simulink model "inverter"  (R2026a)
settings: Solver=VariableStepAuto  StopTime=0.5
libraries: fl_lib x18, nesl_utility x8, ee_lib x2
settings Model: Creator=bilgehan  LastModifiedBy=bilgehan
settings DataIOCC: SaveState=on

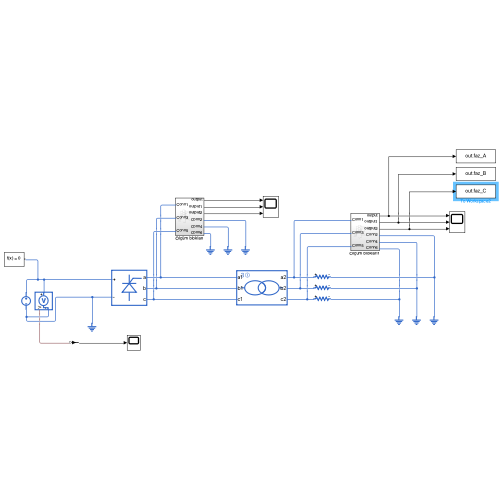
[thumbnail: Simulink's stored preview of the top-level diagram]
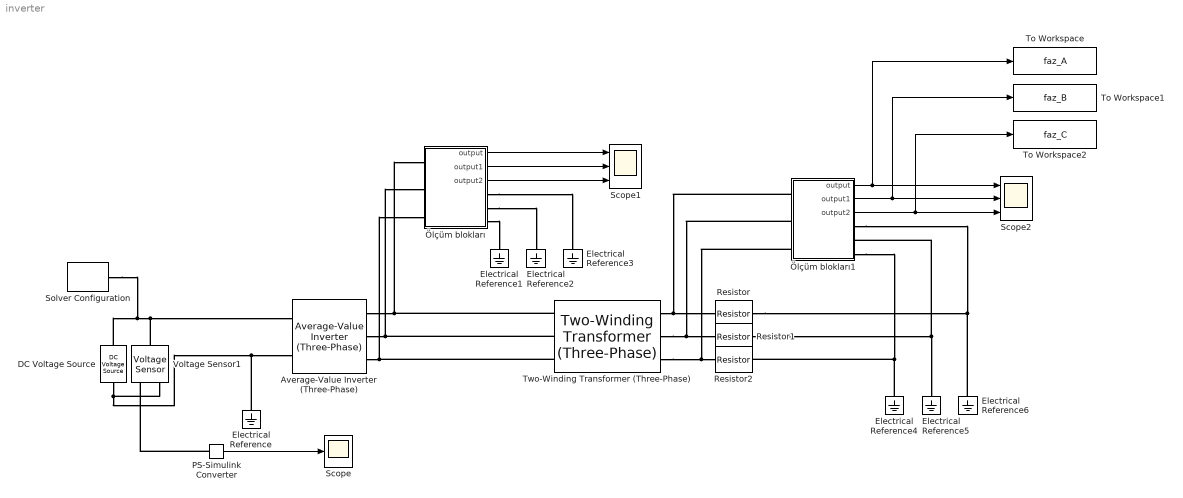
== system inverter ==
  Average-Value Inverter (Three-Phase) : ee_lib/Semiconductors & Converters/Converters/Average-Value Inverter (Three-Phase)  port_option=ee.enum.threePhasePort.expanded  FRated=50 Hz  PhaseShift=0 deg  voltage_ratio=sqrt(6) / pi  Pfixed=1e3 W  v_on=100 V  v_off=75 V
  DC Voltage Source : fl_lib/Electrical/Electrical Sources/DC Voltage Source  v0=400 V
  Electrical Reference{,1..6} (7 alike) : fl_lib/Electrical/Electrical Elements/Electrical Reference
  PS-Simulink Converter : nesl_utility/PS-Simulink Converter  PhysicalDomain=network_engine_domain  SubClassName=ps_output  LeftPortType=input  RightPortType=output  PseudoPeriodic=off  Frequencies=[]  VectorFormat=inherit  Unit=inherit  AffineConversion=off
  Resistor : fl_lib/Electrical/Electrical Elements/Resistor  R=50 Ohm  i_specify=off  i_priority=None  i=0 A  i_nominal_specify=off  i_nominal_value=1  i_nominal_unit=A  v_specify=off  v_priority=None  v=0 V  v_nominal_specify=off  v_nominal_value=1  v_nominal_unit=V
  Resistor1 : fl_lib/Electrical/Electrical Elements/Resistor  R=50 Ohm  i_specify=off  i_priority=None  i=0 A  i_nominal_specify=off  i_nominal_value=1  i_nominal_unit=A  v_specify=off  v_priority=None  v=0 V  v_nominal_specify=off  v_nominal_value=1  v_nominal_unit=V
  Resistor2 : fl_lib/Electrical/Electrical Elements/Resistor  R=50 Ohm  i_specify=off  i_priority=None  i=0 A  i_nominal_specify=off  i_nominal_value=1  i_nominal_unit=A  v_specify=off  v_priority=None  v=0 V  v_nominal_specify=off  v_nominal_value=1  v_nominal_unit=V
  Scope : Scope
      settings: ActiveDisplayYMinimum=-118.30988508385255  ActiveDisplayYMaximum=518.30988605563437
  Scope1 : Scope  NumInputPorts=3
      settings: ActiveDisplayYMinimum=-118.30987454094273  ActiveDisplayYMaximum=518.30988273667788
  Scope2 : Scope  NumInputPorts=3
      settings: ActiveDisplayYMinimum=-402.70817553940793  ActiveDisplayYMaximum=402.70749472920392  DataLoggingVariableName=trafo_out
  Solver Configuration : nesl_utility/Solver Configuration  PhysicalDomain=network_engine_domain  SubClassName=solver  LeftPortType=input  RightPortType=generic  Tones=[]  Harmonics=[]  SimulateNoise=off  Profile=off  UseLocalSampling=off  EnableSwitchedLinearOptims=on  FrequencyDomain=off  UseCCode=off  RelTol=0.001  AbsTol=0.001  MinStep=1e-09  ToWorkspace=off  RevertToSquareIcSolve=off  NumHomotopyIterations=100  PhasorMode=off  PhasorModeNumHarmonics=1  ConsistencySolver=NEWTON_XTOL_AFTER_FTOL  CanonicalOrdering=CANONICAL  OptimizeIntermediates=OPTIMIZED  IndexReductionMethod=DerivativeReplacement  DoDC=off  ResidualTolerance=1e-09  ConsistencyTolSource=GLOBAL  ConsistencyAbsTol=0.001  ConsistencyRelTol=0.001  ConsistencyTolFactor=0.001  UseLocalSolver=off  LocalSolverChoice=NE_BACKWARD_EULER_ADVANCER  ResolveIndetEquations=on  FunctionEvalNumThread=1  LocalSolverSampleTime=0.001  DoFixedCost=off  MaxNonlinIter=3  MaxModeIter=2  ComputeImpulses=off  ImpulseIterations=2  LinearAlgebra=auto  LinearAlgebraNumThread=0  EquationFormulation=NE_TIME_EF  DelaysMemoryBudget=1024  AutomaticFiltering=on  FilteringTimeConstant=0.001  PartitionStorageMethod=AS_NEEDED  PartitionMemoryBudget=1024  PartitionMethod=ROBUST  MultibodyUseLocalSolver=off  MultibodyLocalSolverChoice=ODE1  MultibodyLocalSolverSampleTime=0.001
  To Workspace : ToWorkspace  VariableName=faz_A  SampleTime=-1
  To Workspace1 : ToWorkspace  VariableName=faz_B  SampleTime=-1
  To Workspace2 : ToWorkspace  VariableName=faz_C  SampleTime=-1
  Two-Winding Transformer (Three-Phase) : ee_lib/Passive/Transformers/Two-Winding Transformer (Three-Phase)  SRated=3250 A*V  FRated=50 Hz  Winding1Connection=ee.enum.windingconnection.Y  VRated1=311 V  Winding2Connection=ee.enum.windingconnection.Y  VRated2=400 V  CoreType=ee.enum.coretype.threelimb  pu_Rw1=0.002  pu_Rw2=0.01  leakage_reactance_option=ee.enum.transformer_leakage.include  pu_Xl1=0.05  pu_Xl2=0.05  magnetizing_resistance_option=ee.enum.transformer_magnetizingResistance.exclude  pu_Rm=500  magnetizing_reactance_option=ee.enum.transformer_magnetizingReactance.exclude  saturation_option=ee.enum.transformer_saturation.exclude  pu_Xm=500  current_data=[0, .002, 1, 2]  magnetic_flux_data=[0, 1.2, 1.5, 1.51]  pu_X0=0.5  i1_specify=off  i1_priority=None  i1=[0, 0, 0] A  i1_nominal_specify=off  i1_nominal_value=1  i1_nominal_unit=A  i2_specify=off  i2_priority=None  i2=[0, 0, 0] A  i2_nominal_specify=off  i2_nominal_value=1  i2_nominal_unit=A  phi_specify=off  phi_priority=None  phi=[0, 0, 0]  phi_nominal_specify=off  phi_nominal_value=1  phi_nominal_unit=1
  Voltage Sensor1 : fl_lib/Electrical/Electrical Sensors/Voltage Sensor
  Ölçüm blokları : Subsystem
  Ölçüm blokları1 : Subsystem
  wires:
  PS-Simulink Converter/1 -> Scope/1
  Ölçüm blokları/1(output) -> Scope1/1
  Ölçüm blokları/2(output1) -> Scope1/2
  Ölçüm blokları/3(output2) -> Scope1/3
  Ölçüm blokları1/2(output1) -> To Workspace1/1, Scope2/2
  Ölçüm blokları1/3(output2) -> To Workspace2/1, Scope2/3
  Ölçüm blokları1/1(output) -> To Workspace/1, Scope2/1
  connections:
  DC Voltage Source/LConn1 -- Solver Configuration/RConn1 -- Average-Value Inverter (Three-Phase)/LConn1 -- Voltage Sensor1/LConn1
  DC Voltage Source/RConn1 -- Voltage Sensor1/RConn2 -- Average-Value Inverter (Three-Phase)/LConn2 -- Electrical Reference/LConn1
  Average-Value Inverter (Three-Phase)/RConn1 -- Two-Winding Transformer (Three-Phase)/LConn1 -- Ölçüm blokları/LConn1
  Average-Value Inverter (Three-Phase)/RConn2 -- Two-Winding Transformer (Three-Phase)/LConn2 -- Ölçüm blokları/LConn2
  Average-Value Inverter (Three-Phase)/RConn3 -- Ölçüm blokları/LConn3 -- Two-Winding Transformer (Three-Phase)/LConn3
  PS-Simulink Converter/LConn1 -- Voltage Sensor1/RConn1
  Ölçüm blokları/RConn3 -- Electrical Reference1/LConn1
  Ölçüm blokları/RConn2 -- Electrical Reference2/LConn1
  Ölçüm blokları/RConn1 -- Electrical Reference3/LConn1
  Two-Winding Transformer (Three-Phase)/RConn1 -- Ölçüm blokları1/LConn1 -- Resistor/LConn1
  Two-Winding Transformer (Three-Phase)/RConn2 -- Ölçüm blokları1/LConn2 -- Resistor1/LConn1
  Two-Winding Transformer (Three-Phase)/RConn3 -- Ölçüm blokları1/LConn3 -- Resistor2/LConn1
  Electrical Reference4/LConn1 -- Ölçüm blokları1/RConn3 -- Resistor2/RConn1
  Resistor/RConn1 -- Ölçüm blokları1/RConn1 -- Electrical Reference6/LConn1
  Resistor1/RConn1 -- Ölçüm blokları1/RConn2 -- Electrical Reference5/LConn1

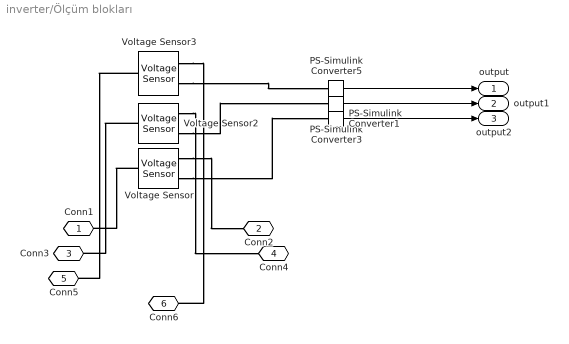
== system inverter/Ölçüm blokları ==
  PS-Simulink Converter1 : nesl_utility/PS-Simulink Converter  PhysicalDomain=network_engine_domain  SubClassName=ps_output  LeftPortType=input  RightPortType=output  PseudoPeriodic=off  Frequencies=[]  VectorFormat=inherit  Unit=inherit  AffineConversion=off
  PS-Simulink Converter3 : nesl_utility/PS-Simulink Converter  PhysicalDomain=network_engine_domain  SubClassName=ps_output  LeftPortType=input  RightPortType=output  PseudoPeriodic=off  Frequencies=[]  VectorFormat=inherit  Unit=inherit  AffineConversion=off
  PS-Simulink Converter5 : nesl_utility/PS-Simulink Converter  PhysicalDomain=network_engine_domain  SubClassName=ps_output  LeftPortType=input  RightPortType=output  PseudoPeriodic=off  Frequencies=[]  VectorFormat=inherit  Unit=inherit  AffineConversion=off
  Voltage Sensor : fl_lib/Electrical/Electrical Sensors/Voltage Sensor
  Voltage Sensor2 : fl_lib/Electrical/Electrical Sensors/Voltage Sensor
  Voltage Sensor3 : fl_lib/Electrical/Electrical Sensors/Voltage Sensor
  Conn1 : PMIOPort  Side=Left
  Conn2 : PMIOPort  Port=2  Side=Right
  Conn3 : PMIOPort  Port=3  Side=Left
  Conn4 : PMIOPort  Port=4  Side=Right
  Conn5 : PMIOPort  Port=5  Side=Left
  Conn6 : PMIOPort  Port=6  Side=Right
  output : Outport
  output1 : Outport  Port=2
  output2 : Outport  Port=3
  wires:
  PS-Simulink Converter1/1 -> output2/1
  PS-Simulink Converter3/1 -> output1/1
  PS-Simulink Converter5/1 -> output/1
  connections:
  Voltage Sensor/RConn1 -- PS-Simulink Converter1/LConn1
  Voltage Sensor/LConn1 -- Conn1/RConn1
  Voltage Sensor2/LConn1 -- Conn3/RConn1
  Voltage Sensor3/LConn1 -- Conn5/RConn1
  Voltage Sensor2/RConn2 -- Conn4/RConn1
  Voltage Sensor/RConn2 -- Conn2/RConn1
  Voltage Sensor3/RConn2 -- Conn6/RConn1
  Voltage Sensor3/RConn1 -- PS-Simulink Converter5/LConn1
  Voltage Sensor2/RConn1 -- PS-Simulink Converter3/LConn1

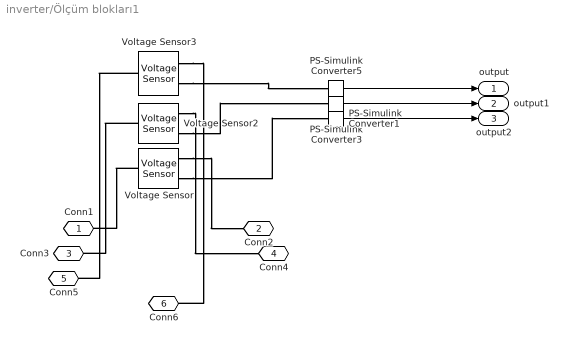
== system inverter/Ölçüm blokları1 ==
  PS-Simulink Converter1 : nesl_utility/PS-Simulink Converter  PhysicalDomain=network_engine_domain  SubClassName=ps_output  LeftPortType=input  RightPortType=output  PseudoPeriodic=off  Frequencies=[]  VectorFormat=inherit  Unit=inherit  AffineConversion=off
  PS-Simulink Converter3 : nesl_utility/PS-Simulink Converter  PhysicalDomain=network_engine_domain  SubClassName=ps_output  LeftPortType=input  RightPortType=output  PseudoPeriodic=off  Frequencies=[]  VectorFormat=inherit  Unit=inherit  AffineConversion=off
  PS-Simulink Converter5 : nesl_utility/PS-Simulink Converter  PhysicalDomain=network_engine_domain  SubClassName=ps_output  LeftPortType=input  RightPortType=output  PseudoPeriodic=off  Frequencies=[]  VectorFormat=inherit  Unit=inherit  AffineConversion=off
  Voltage Sensor : fl_lib/Electrical/Electrical Sensors/Voltage Sensor
  Voltage Sensor2 : fl_lib/Electrical/Electrical Sensors/Voltage Sensor
  Voltage Sensor3 : fl_lib/Electrical/Electrical Sensors/Voltage Sensor
  Conn1 : PMIOPort  Side=Left
  Conn2 : PMIOPort  Port=2  Side=Right
  Conn3 : PMIOPort  Port=3  Side=Left
  Conn4 : PMIOPort  Port=4  Side=Right
  Conn5 : PMIOPort  Port=5  Side=Left
  Conn6 : PMIOPort  Port=6  Side=Right
  output : Outport
  output1 : Outport  Port=2
  output2 : Outport  Port=3
  wires:
  PS-Simulink Converter1/1 -> output2/1
  PS-Simulink Converter3/1 -> output1/1
  PS-Simulink Converter5/1 -> output/1
  connections:
  Voltage Sensor/RConn1 -- PS-Simulink Converter1/LConn1
  Voltage Sensor/LConn1 -- Conn1/RConn1
  Voltage Sensor2/LConn1 -- Conn3/RConn1
  Voltage Sensor3/LConn1 -- Conn5/RConn1
  Voltage Sensor2/RConn2 -- Conn4/RConn1
  Voltage Sensor/RConn2 -- Conn2/RConn1
  Voltage Sensor3/RConn2 -- Conn6/RConn1
  Voltage Sensor3/RConn1 -- PS-Simulink Converter5/LConn1
  Voltage Sensor2/RConn1 -- PS-Simulink Converter3/LConn1
